simulink model "atrias_system_4khz_with_boom"  (R2016b)
settings: configuration reference "Configuration4khz" (kept outside this file)
undefined symbols (not defined in the file or in its folder): BOOM_MAX_ENCODER_TICKS, elmo_sample_time, gui_disable_cmd, gui_enable_cmd, gui_exit_cmd, gui_reset_cmd, HARD_MOTOR_POSITION_LIMITS_LOWER, HARD_MOTOR_POSITION_LIMITS_UPPER, HIP_ABS_MAX_ENCODER_TICKS, HIP_CURRENT_LIMIT, HIP_INC_MAX_ENCODER_TICKS, HIP_MOTOR_CONSTANT, HIP_MTR_GEAR_RATIO, HIP_MTR_MAX_TORQUE, LEFT_MOTOR_HIP_DIRECTION, LEG1_MOTOR_A_DIRECTION, LEG1_MOTOR_B_DIRECTION, LEG2_MOTOR_A_DIRECTION, LEG2_MOTOR_B_DIRECTION, LEG_CURRENT_LIMIT, LEG_INC_ENCODER_DIRECTION_LEFT_BACK, LEG_INC_ENCODER_DIRECTION_LEFT_FRONT, LEG_INC_ENCODER_DIRECTION_RIGHT_BACK, LEG_INC_ENCODER_DIRECTION_RIGHT_FRONT, LEG_INC_ENCODER_RAD_PER_TICK, LEG_MOTOR_CONSTANT, LEG_MTR_GEAR_RATIO, LEG_MTR_MAX_TORQUE, max_hip_velocity, max_motor_velocity, MEDULLA_ADC_MAX_VOLTS, MEDULLA_ADC_OFFSET_COUNTS, MEDULLA_STATE_ERROR, MEDULLA_STATE_HALT, MEDULLA_STATE_IDLE, MEDULLA_STATE_RESET, MEDULLA_STATE_RUN, MOTOR_POSITION_LIMITS_LOWER, MOTOR_POSITION_LIMITS_UPPER, MTR_HIP_MAX_CURRENT, MTR_MAX_CONT_CURRENT, MTR_MAX_COUNT, MTR_MAX_CURRENT, MTR_MAX_TEMP, RIGHT_MOTOR_HIP_DIRECTION
libraries: xpcethercatlib x203, simulink x38
(part 2 of 4)

== system atrias_system_4khz_with_boom/Ramp Velocity Commands ==
  note: For GUI
  is_run_cmd : Inport  OutDataTypeStr=boolean  PortDimensions=1
  system time [s] : Inport  Port=2  PortDimensions=1
  velocity_cmd [rad/s] x4 : Inport  Port=3
  Constant : Constant  Value=0.1
  Enabled time : Sum  Inputs=-+
  Hold Start Time : Subsystem  TreatAsAtomicUnit=on
  NOT : Logic  Operator=NOT  IconShape=distinctive  AllPortsSameDT=off  OutDataTypeStr=boolean
  Ramp Rate (Units/sec) : Gain  Gain=1/4
  Scaling Factor : Saturate  UpperLimit=1  LowerLimit=0
  Startup Ramp : Product
  Sum : Sum  Inputs=|-+
  Terminator : Terminator
  is_start_done_cmp : RelationalOperator  Operator=>  OutDataTypeStr=boolean  RndMeth=Nearest
  velocity_cmd_scaled [rad/s] x4 : Outport  OutDataTypeStr=double  PortDimensions=4
  wires:
  is_start_done_cmp/1 -> Terminator/1
  Sum/1 -> is_start_done_cmp/1
  velocity_cmd [rad/s] x4/1 -> Startup Ramp/2
  Startup Ramp/1 -> velocity_cmd_scaled [rad/s] x4/1
  Scaling Factor/1 -> Startup Ramp/1, is_start_done_cmp/2
  Ramp Rate (Units/sec)/1 -> Sum/2, Scaling Factor/1
  Enabled time/1 -> Ramp Rate (Units/sec)/1
  Hold Start Time/1(Time Out) -> Enabled time/1
  system time [s]/1 -> Enabled time/2, Hold Start Time/1(Time In)
  is_run_cmd/1 -> NOT/1
  NOT/1 -> Hold Start Time/Enable
  Constant/1 -> Sum/1

== system atrias_system_4khz_with_boom/Start Controller ==
  note: For GUI
  note: Input Order:
      |
      | backR
      | frontR
      | latR
      | backL
      | frontL
      | latL
  is_run_cmd : Inport  OutDataTypeStr=boolean  PortDimensions=1
  system time [s] : Inport  Port=2  PortDimensions=1
  tau_cmd_in [Nm] x6 : Inport  Port=3
  Enabled time : Sum  Inputs=-+
  Hold Start Time : Subsystem  TreatAsAtomicUnit=on
  Lateral Motor Saturation : Saturate  UpperLimit=HIP_MTR_MAX_TORQUE  LowerLimit=-HIP_MTR_MAX_TORQUE
      settings: AttributesFormatString=Top: %<UpperLimit>\nBottom: %<LowerLimit>
  NOT : Logic  Operator=NOT  IconShape=distinctive  AllPortsSameDT=off  OutDataTypeStr=boolean
  Ramp Rate (Units/sec) : Gain  Gain=.25
  Sagittal Motor Saturation : Saturate  UpperLimit=LEG_MTR_MAX_TORQUE  LowerLimit=-LEG_MTR_MAX_TORQUE
      settings: AttributesFormatString=Top: %<UpperLimit>\nBottom: %<LowerLimit>
  Scaling Factor : Saturate  UpperLimit=1  LowerLimit=0
  Selector : Selector  InputPortWidth=6  IndexOptions=Index vector (dialog)  Indices=[1 2 4 5 6 3]  OutputSizes=1
  Selector1 : Selector  InputPortWidth=6  IndexOptions=Index vector (dialog)  Indices=[1 2 3 4]  OutputSizes=1
  Selector2 : Selector  InputPortWidth=6  IndexOptions=Index vector (dialog)  Indices=[5 6]  OutputSizes=1
  Separated to Tau : Selector  InputPortWidth=6  IndexOptions=Index vector (dialog)  Indices=[1 2 6 3 4 5]  OutputSizes=1
  Startup Tau Ramp : Product
  Sum : Sum  Inputs=|-+
  Terminator : Terminator
  Vector Concatenate : Concatenate
  is_start_done_cmp : RelationalOperator  Operator=>  OutDataTypeStr=boolean  RndMeth=Nearest
  tau_cmd_out [Nm] x6 : Outport  OutDataTypeStr=double  PortDimensions=6
  wires:
  NOT/1 -> Hold Start Time/Enable
  is_run_cmd/1 -> NOT/1
  system time [s]/1 -> Enabled time/2, Hold Start Time/1(Time In)
  Hold Start Time/1(Time Out) -> Enabled time/1
  Enabled time/1 -> Ramp Rate (Units/sec)/1
  Ramp Rate (Units/sec)/1 -> Scaling Factor/1, Sum/2
  Scaling Factor/1 -> is_start_done_cmp/2, Startup Tau Ramp/1
  Startup Tau Ramp/1 -> tau_cmd_out [Nm] x6/1
  Selector2/1 -> Lateral Motor Saturation/1  "lateral"
  Selector1/1 -> Sagittal Motor Saturation/1  "sagittal"
  tau_cmd_in [Nm] x6/1 -> Selector/1
  Selector/1 -> Selector1/1, Selector2/1
  Sagittal Motor Saturation/1 -> Vector Concatenate/1
  Lateral Motor Saturation/1 -> Vector Concatenate/2
  Vector Concatenate/1 -> Separated to Tau/1
  Separated to Tau/1 -> Startup Tau Ramp/2
  Sum/1 -> is_start_done_cmp/1
  is_start_done_cmp/1 -> Terminator/1

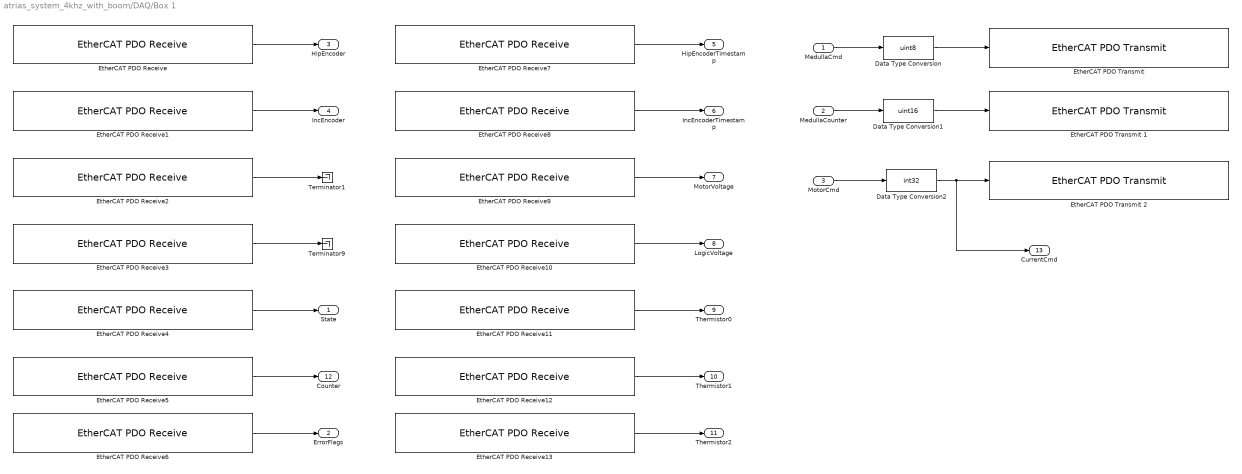
== system atrias_system_4khz_with_boom/DAQ/Box 1 ==
  MedullaCmd : Inport
  MedullaCounter : Inport  Port=2
  MotorCmd : Inport  Port=3
  Data Type Conversion : DataTypeConversion  OutDataTypeStr=uint8
  Data Type Conversion1 : DataTypeConversion  OutDataTypeStr=uint16
  Data Type Conversion2 : DataTypeConversion  OutDataTypeStr=int32
  EtherCAT PDO Receive : xpcethercatlib/EtherCAT PDO Receive  Priority=2  sig_name=Box 1 (ATRIAS 2.1 Hip (Medulla 1.5)).Hip Encoder.Encoder  sig_offset=504  sig_type=uint32  type_size=32  sig_dim=1  device_id=0  sample_time=0.001000
  EtherCAT PDO Receive1 : xpcethercatlib/EtherCAT PDO Receive  Priority=2  sig_name=Box 1 (ATRIAS 2.1 Hip (Medulla 1.5)).Incremental Encoder.Incremental Encoder  sig_offset=648  sig_type=uint16  type_size=16  sig_dim=1  device_id=0  sample_time=0.001000
  EtherCAT PDO Receive10 : xpcethercatlib/EtherCAT PDO Receive  Priority=2  sig_name=Box 1 (ATRIAS 2.1 Hip (Medulla 1.5)).Power.Logic Voltage  sig_offset=568  sig_type=uint16  type_size=16  sig_dim=1  device_id=0  sample_time=0.001000
  EtherCAT PDO Receive11 : xpcethercatlib/EtherCAT PDO Receive  Priority=2  sig_name=Box 1 (ATRIAS 2.1 Hip (Medulla 1.5)).Thermistors.Thermistor 0  sig_offset=584  sig_type=uint16  type_size=16  sig_dim=1  device_id=0  sample_time=0.001000
  EtherCAT PDO Receive12 : xpcethercatlib/EtherCAT PDO Receive  Priority=2  sig_name=Box 1 (ATRIAS 2.1 Hip (Medulla 1.5)).Thermistors.Thermistor 1  sig_offset=600  sig_type=uint16  type_size=16  sig_dim=1  device_id=0  sample_time=0.001000
  EtherCAT PDO Receive13 : xpcethercatlib/EtherCAT PDO Receive  Priority=2  sig_name=Box 1 (ATRIAS 2.1 Hip (Medulla 1.5)).Thermistors.Thermistor 2  sig_offset=616  sig_type=uint16  type_size=16  sig_dim=1  device_id=0  sample_time=0.001000
  EtherCAT PDO Receive2 : xpcethercatlib/EtherCAT PDO Receive  Priority=2  sig_name=Box 1 (ATRIAS 2.1 Hip (Medulla 1.5)).uController Status.Limit Switch  sig_offset=496  sig_type=uint8  type_size=8  sig_dim=1  device_id=0  sample_time=0.001000
  EtherCAT PDO Receive3 : xpcethercatlib/EtherCAT PDO Receive  Priority=2  sig_name=Box 1 (ATRIAS 2.1 Hip (Medulla 1.5)).uController Status.ID  sig_offset=464  sig_type=uint8  type_size=8  sig_dim=1  device_id=0  sample_time=0.001000
  EtherCAT PDO Receive4 : xpcethercatlib/EtherCAT PDO Receive  Priority=2  sig_name=Box 1 (ATRIAS 2.1 Hip (Medulla 1.5)).uController Status.State  sig_offset=472  sig_type=uint8  type_size=8  sig_dim=1  device_id=0  sample_time=0.001000
  EtherCAT PDO Receive5 : xpcethercatlib/EtherCAT PDO Receive  Priority=2  sig_name=Box 1 (ATRIAS 2.1 Hip (Medulla 1.5)).uController Status.Counter  sig_offset=480  sig_type=uint8  type_size=8  sig_dim=1  device_id=0  sample_time=0.001000
  EtherCAT PDO Receive6 : xpcethercatlib/EtherCAT PDO Receive  Priority=2  sig_name=Box 1 (ATRIAS 2.1 Hip (Medulla 1.5)).uController Status.Error Flags  sig_offset=488  sig_type=uint8  type_size=8  sig_dim=1  device_id=0  sample_time=0.001000
  EtherCAT PDO Receive7 : xpcethercatlib/EtherCAT PDO Receive  Priority=2  sig_name=Box 1 (ATRIAS 2.1 Hip (Medulla 1.5)).Hip Encoder.Timestamp  sig_offset=536  sig_type=uint16  type_size=16  sig_dim=1  device_id=0  sample_time=0.001000
  EtherCAT PDO Receive8 : xpcethercatlib/EtherCAT PDO Receive  Priority=2  sig_name=Box 1 (ATRIAS 2.1 Hip (Medulla 1.5)).Incremental Encoder.Incremental Encoder Timestamp  sig_offset=664  sig_type=uint16  type_size=16  sig_dim=1  device_id=0  sample_time=0.001000
  EtherCAT PDO Receive9 : xpcethercatlib/EtherCAT PDO Receive  Priority=2  sig_name=Box 1 (ATRIAS 2.1 Hip (Medulla 1.5)).Power.Motor Voltage  sig_offset=552  sig_type=uint16  type_size=16  sig_dim=1  device_id=0  sample_time=0.001000
  "EtherCAT PDO Transmit " : xpcethercatlib/EtherCAT PDO Transmit   Priority=3  sig_name=Box 1 (ATRIAS 2.1 Hip (Medulla 1.5)).uControllerInput.Command  sig_offset=464  sig_type=uint8  type_size=8  sig_dim=1  device_id=0  sample_time=0.001000
  EtherCAT PDO Transmit 1 : xpcethercatlib/EtherCAT PDO Transmit   Priority=3  sig_name=Box 1 (ATRIAS 2.1 Hip (Medulla 1.5)).uControllerInput.Counter  sig_offset=472  sig_type=uint16  type_size=16  sig_dim=1  device_id=0  sample_time=0.001000
  EtherCAT PDO Transmit 2 : xpcethercatlib/EtherCAT PDO Transmit   Priority=3  sig_name=Box 1 (ATRIAS 2.1 Hip (Medulla 1.5)).uControllerInput.Motor Current  sig_offset=488  sig_type=int32  type_size=32  sig_dim=1  device_id=0  sample_time=0.001000
  Terminator1 : Terminator
  Terminator9 : Terminator
  State : Outport
  ErrorFlags : Outport  Port=2
  HipEncoder : Outport  Port=3
  IncEncoder : Outport  Port=4
  HipEncoderTimestamp : Outport  Port=5
  IncEncoderTimestamp : Outport  Port=6
  MotorVoltage : Outport  Port=7
  LogicVoltage : Outport  Port=8
  Thermistor0 : Outport  Port=9
  Thermistor1 : Outport  Port=10
  Thermistor2 : Outport  Port=11
  Counter : Outport  Port=12
  CurrentCmd : Outport  Port=13
  wires:
  Data Type Conversion/1 -> "EtherCAT PDO Transmit "/1
  Data Type Conversion1/1 -> EtherCAT PDO Transmit 1/1
  Data Type Conversion2/1 -> CurrentCmd/1, EtherCAT PDO Transmit 2/1
  MedullaCmd/1 -> Data Type Conversion/1
  MedullaCounter/1 -> Data Type Conversion1/1
  MotorCmd/1 -> Data Type Conversion2/1
  EtherCAT PDO Receive8/1 -> IncEncoderTimestamp/1
  EtherCAT PDO Receive/1 -> HipEncoder/1
  EtherCAT PDO Receive7/1 -> HipEncoderTimestamp/1
  EtherCAT PDO Receive1/1 -> IncEncoder/1
  EtherCAT PDO Receive5/1 -> Counter/1
  EtherCAT PDO Receive3/1 -> Terminator9/1
  EtherCAT PDO Receive4/1 -> State/1
  EtherCAT PDO Receive6/1 -> ErrorFlags/1
  EtherCAT PDO Receive10/1 -> LogicVoltage/1
  EtherCAT PDO Receive9/1 -> MotorVoltage/1
  EtherCAT PDO Receive11/1 -> Thermistor0/1
  EtherCAT PDO Receive12/1 -> Thermistor1/1
  EtherCAT PDO Receive13/1 -> Thermistor2/1
  EtherCAT PDO Receive2/1 -> Terminator1/1

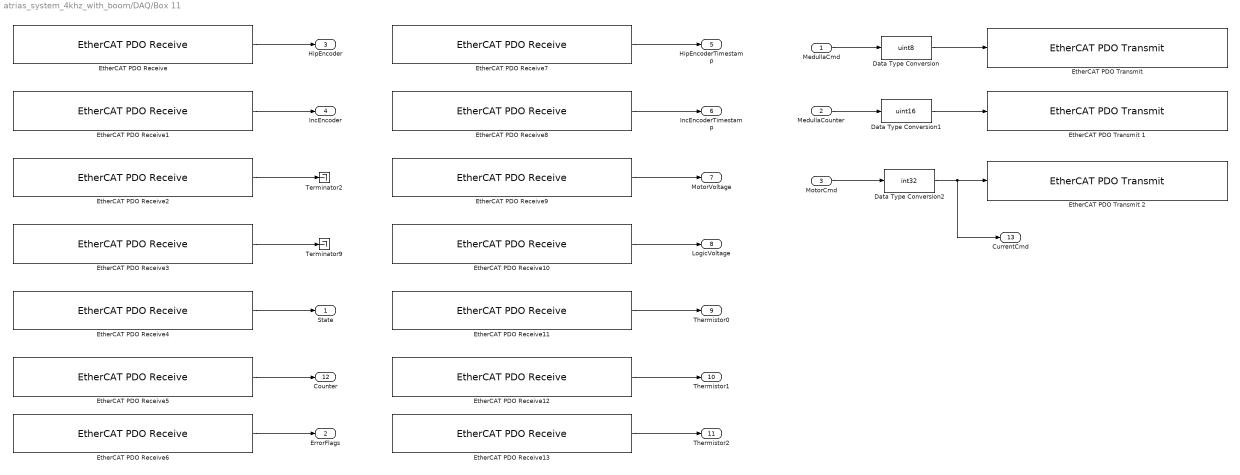
== system atrias_system_4khz_with_boom/DAQ/Box 11 ==
  MedullaCmd : Inport
  MedullaCounter : Inport  Port=2
  MotorCmd : Inport  Port=3
  Data Type Conversion : DataTypeConversion  OutDataTypeStr=uint8
  Data Type Conversion1 : DataTypeConversion  OutDataTypeStr=uint16
  Data Type Conversion2 : DataTypeConversion  OutDataTypeStr=int32
  EtherCAT PDO Receive : xpcethercatlib/EtherCAT PDO Receive  Priority=2  sig_name=Box 11 (ATRIAS 2.1 Hip (Medulla 1.5)).Hip Encoder.Encoder  sig_offset=2512  sig_type=uint32  type_size=32  sig_dim=1  device_id=0  sample_time=0.001000
  EtherCAT PDO Receive1 : xpcethercatlib/EtherCAT PDO Receive  Priority=2  sig_name=Box 11 (ATRIAS 2.1 Hip (Medulla 1.5)).Incremental Encoder.Incremental Encoder  sig_offset=2656  sig_type=uint16  type_size=16  sig_dim=1  device_id=0  sample_time=0.001000
  EtherCAT PDO Receive10 : xpcethercatlib/EtherCAT PDO Receive  Priority=2  sig_name=Box 11 (ATRIAS 2.1 Hip (Medulla 1.5)).Power.Logic Voltage  sig_offset=2576  sig_type=uint16  type_size=16  sig_dim=1  device_id=0  sample_time=0.001000
  EtherCAT PDO Receive11 : xpcethercatlib/EtherCAT PDO Receive  Priority=2  sig_name=Box 11 (ATRIAS 2.1 Hip (Medulla 1.5)).Thermistors.Thermistor 0  sig_offset=2592  sig_type=uint16  type_size=16  sig_dim=1  device_id=0  sample_time=0.001000
  EtherCAT PDO Receive12 : xpcethercatlib/EtherCAT PDO Receive  Priority=2  sig_name=Box 11 (ATRIAS 2.1 Hip (Medulla 1.5)).Thermistors.Thermistor 1  sig_offset=2608  sig_type=uint16  type_size=16  sig_dim=1  device_id=0  sample_time=0.001000
  EtherCAT PDO Receive13 : xpcethercatlib/EtherCAT PDO Receive  Priority=2  sig_name=Box 11 (ATRIAS 2.1 Hip (Medulla 1.5)).Thermistors.Thermistor 2  sig_offset=2624  sig_type=uint16  type_size=16  sig_dim=1  device_id=0  sample_time=0.001000
  EtherCAT PDO Receive2 : xpcethercatlib/EtherCAT PDO Receive  Priority=2  sig_name=Box 11 (ATRIAS 2.1 Hip (Medulla 1.5)).uController Status.Limit Switch  sig_offset=2504  sig_type=uint8  type_size=8  sig_dim=1  device_id=0  sample_time=0.001000
  EtherCAT PDO Receive3 : xpcethercatlib/EtherCAT PDO Receive  Priority=2  sig_name=Box 11 (ATRIAS 2.1 Hip (Medulla 1.5)).uController Status.ID  sig_offset=2472  sig_type=uint8  type_size=8  sig_dim=1  device_id=0  sample_time=0.001000
  EtherCAT PDO Receive4 : xpcethercatlib/EtherCAT PDO Receive  Priority=2  sig_name=Box 11 (ATRIAS 2.1 Hip (Medulla 1.5)).uController Status.State  sig_offset=2480  sig_type=uint8  type_size=8  sig_dim=1  device_id=0  sample_time=0.001000
  EtherCAT PDO Receive5 : xpcethercatlib/EtherCAT PDO Receive  Priority=2  sig_name=Box 11 (ATRIAS 2.1 Hip (Medulla 1.5)).uController Status.Counter  sig_offset=2488  sig_type=uint8  type_size=8  sig_dim=1  device_id=0  sample_time=0.001000
  EtherCAT PDO Receive6 : xpcethercatlib/EtherCAT PDO Receive  Priority=2  sig_name=Box 11 (ATRIAS 2.1 Hip (Medulla 1.5)).uController Status.Error Flags  sig_offset=2496  sig_type=uint8  type_size=8  sig_dim=1  device_id=0  sample_time=0.001000
  EtherCAT PDO Receive7 : xpcethercatlib/EtherCAT PDO Receive  Priority=2  sig_name=Box 11 (ATRIAS 2.1 Hip (Medulla 1.5)).Hip Encoder.Timestamp  sig_offset=2544  sig_type=uint16  type_size=16  sig_dim=1  device_id=0  sample_time=0.001000
  EtherCAT PDO Receive8 : xpcethercatlib/EtherCAT PDO Receive  Priority=2  sig_name=Box 11 (ATRIAS 2.1 Hip (Medulla 1.5)).Incremental Encoder.Incremental Encoder Timestamp  sig_offset=2672  sig_type=uint16  type_size=16  sig_dim=1  device_id=0  sample_time=0.001000
  EtherCAT PDO Receive9 : xpcethercatlib/EtherCAT PDO Receive  Priority=2  sig_name=Box 11 (ATRIAS 2.1 Hip (Medulla 1.5)).Power.Motor Voltage  sig_offset=2560  sig_type=uint16  type_size=16  sig_dim=1  device_id=0  sample_time=0.001000
  EtherCAT PDO Transmit : xpcethercatlib/EtherCAT PDO Transmit   Priority=3  sig_name=Box 11 (ATRIAS 2.1 Hip (Medulla 1.5)).uControllerInput.Command  sig_offset=2472  sig_type=uint8  type_size=8  sig_dim=1  device_id=0  sample_time=0.001000
  "EtherCAT PDO Transmit 1 " : xpcethercatlib/EtherCAT PDO Transmit   Priority=3  sig_name=Box 11 (ATRIAS 2.1 Hip (Medulla 1.5)).uControllerInput.Counter  sig_offset=2480  sig_type=uint16  type_size=16  sig_dim=1  device_id=0  sample_time=0.001000
  EtherCAT PDO Transmit 2 : xpcethercatlib/EtherCAT PDO Transmit   Priority=3  sig_name=Box 11 (ATRIAS 2.1 Hip (Medulla 1.5)).uControllerInput.Motor Current  sig_offset=2496  sig_type=int32  type_size=32  sig_dim=1  device_id=0  sample_time=0.001000
  Terminator2 : Terminator
  Terminator9 : Terminator
  State : Outport
  ErrorFlags : Outport  Port=2
  HipEncoder : Outport  Port=3
  IncEncoder : Outport  Port=4
  HipEncoderTimestamp : Outport  Port=5
  IncEncoderTimestamp : Outport  Port=6
  MotorVoltage : Outport  Port=7
  LogicVoltage : Outport  Port=8
  Thermistor0 : Outport  Port=9
  Thermistor1 : Outport  Port=10
  Thermistor2 : Outport  Port=11
  Counter : Outport  Port=12
  CurrentCmd : Outport  Port=13
  wires:
  Data Type Conversion/1 -> EtherCAT PDO Transmit/1
  Data Type Conversion1/1 -> "EtherCAT PDO Transmit 1 "/1
  Data Type Conversion2/1 -> CurrentCmd/1, EtherCAT PDO Transmit 2/1
  MedullaCmd/1 -> Data Type Conversion/1
  MedullaCounter/1 -> Data Type Conversion1/1
  MotorCmd/1 -> Data Type Conversion2/1
  EtherCAT PDO Receive8/1 -> IncEncoderTimestamp/1
  EtherCAT PDO Receive/1 -> HipEncoder/1
  EtherCAT PDO Receive7/1 -> HipEncoderTimestamp/1
  EtherCAT PDO Receive1/1 -> IncEncoder/1
  EtherCAT PDO Receive5/1 -> Counter/1
  EtherCAT PDO Receive3/1 -> Terminator9/1
  EtherCAT PDO Receive2/1 -> Terminator2/1
  EtherCAT PDO Receive4/1 -> State/1
  EtherCAT PDO Receive6/1 -> ErrorFlags/1
  EtherCAT PDO Receive10/1 -> LogicVoltage/1
  EtherCAT PDO Receive9/1 -> MotorVoltage/1
  EtherCAT PDO Receive11/1 -> Thermistor0/1
  EtherCAT PDO Receive12/1 -> Thermistor1/1
  EtherCAT PDO Receive13/1 -> Thermistor2/1

== system atrias_system_4khz_with_boom/DAQ/Box 2 ==
  MedullaCmd : Inport
  MedullaCounter : Inport  Port=2
  Data Type Conversion : DataTypeConversion  OutDataTypeStr=uint8
  Data Type Conversion1 : DataTypeConversion  OutDataTypeStr=uint16
  EtherCAT PDO Receive1 : xpcethercatlib/EtherCAT PDO Receive  Priority=2  sig_name=Box 12 (ATRIAS 2.1 Boom (Medulla 1.5)).X Encoder.Encoder  sig_offset=2848  sig_type=uint32  type_size=32  sig_dim=1  device_id=0  sample_time=0.001
  EtherCAT PDO Receive13 : xpcethercatlib/EtherCAT PDO Receive  Priority=2  sig_name=Box 12 (ATRIAS 2.1 Boom (Medulla 1.5)).uController Status.Counter  sig_offset=2832  sig_type=uint8  type_size=8  sig_dim=1  device_id=0  sample_time=0.001
  EtherCAT PDO Receive2 : xpcethercatlib/EtherCAT PDO Receive  Priority=2  sig_name=Box 12 (ATRIAS 2.1 Boom (Medulla 1.5)).Z Encoder.Encoder  sig_offset=2944  sig_type=uint32  type_size=32  sig_dim=1  device_id=0  sample_time=0.001
  EtherCAT PDO Receive3 : xpcethercatlib/EtherCAT PDO Receive  Priority=2  sig_name=Box 12 (ATRIAS 2.1 Boom (Medulla 1.5)).X Encoder.Timestamp  sig_offset=2880  sig_type=uint16  type_size=16  sig_dim=1  device_id=0  sample_time=0.001
  EtherCAT PDO Receive4 : xpcethercatlib/EtherCAT PDO Receive  Priority=2  sig_name=Box 12 (ATRIAS 2.1 Boom (Medulla 1.5)).Pitch Encoder.Encoder  sig_offset=2896  sig_type=uint32  type_size=32  sig_dim=1  device_id=0  sample_time=0.001
  EtherCAT PDO Receive5 : xpcethercatlib/EtherCAT PDO Receive  Priority=2  sig_name=Box 12 (ATRIAS 2.1 Boom (Medulla 1.5)).Z Encoder.Timestamp  sig_offset=2976  sig_type=uint16  type_size=16  sig_dim=1  device_id=0  sample_time=0.001
  EtherCAT PDO Receive6 : xpcethercatlib/EtherCAT PDO Receive  Priority=2  sig_name=Box 12 (ATRIAS 2.1 Boom (Medulla 1.5)).Pitch Encoder.Timestamp  sig_offset=2928  sig_type=uint16  type_size=16  sig_dim=1  device_id=0  sample_time=0.001
  EtherCAT PDO Transmit : xpcethercatlib/EtherCAT PDO Transmit   Priority=3  sig_name=Box 12 (ATRIAS 2.1 Boom (Medulla 1.5)).uControllerInput.Command  sig_offset=2816  sig_type=uint8  type_size=8  sig_dim=1  device_id=0  sample_time=0.001
  EtherCAT PDO Transmit1 : xpcethercatlib/EtherCAT PDO Transmit   Priority=3  sig_name=Box 12 (ATRIAS 2.1 Boom (Medulla 1.5)).uControllerInput.Counter  sig_offset=2824  sig_type=uint16  type_size=16  sig_dim=1  device_id=0  sample_time=0.001
  Pitch Encoder : Outport
  X Encoder : Outport  Port=2
  Z Encoder : Outport  Port=3
  Pitch Encoder Timestamp : Outport  Port=4
  X Encoder Timestamp : Outport  Port=5
  Z Encoder Timestamp : Outport  Port=6
  Counter : Outport  Port=7
  wires:
  EtherCAT PDO Receive13/1 -> Counter/1
  Data Type Conversion/1 -> EtherCAT PDO Transmit/1
  Data Type Conversion1/1 -> EtherCAT PDO Transmit1/1
  MedullaCmd/1 -> Data Type Conversion/1
  MedullaCounter/1 -> Data Type Conversion1/1
  EtherCAT PDO Receive4/1 -> Pitch Encoder/1
  EtherCAT PDO Receive1/1 -> X Encoder/1
  EtherCAT PDO Receive2/1 -> Z Encoder/1
  EtherCAT PDO Receive6/1 -> Pitch Encoder Timestamp/1
  EtherCAT PDO Receive3/1 -> X Encoder Timestamp/1
  EtherCAT PDO Receive5/1 -> Z Encoder Timestamp/1

== system atrias_system_4khz_with_boom/DAQ/Box 4 ==
  MedullaCmd : Inport
  MedullaCounter : Inport  Port=2
  Data Type Conversion : DataTypeConversion  OutDataTypeStr=uint8
  Data Type Conversion1 : DataTypeConversion  OutDataTypeStr=uint16
  EtherCAT PDO Receive1 : xpcethercatlib/EtherCAT PDO Receive  Priority=2  sig_name=Box 4 (ATRIAS 2.1 IMU (Medulla 1.5)).Rotation.Y  sig_offset=776  sig_type=single  type_size=32  sig_dim=1  device_id=0  sample_time=0.001000
  EtherCAT PDO Receive11 : xpcethercatlib/EtherCAT PDO Receive  Priority=2  sig_name=Box 4 (ATRIAS 2.1 IMU (Medulla 1.5)).uController Status.ID  sig_offset=712  sig_type=uint8  type_size=8  sig_dim=1  device_id=0  sample_time=0.001000
  EtherCAT PDO Receive12 : xpcethercatlib/EtherCAT PDO Receive  Priority=2  sig_name=Box 4 (ATRIAS 2.1 IMU (Medulla 1.5)).uController Status.State  sig_offset=720  sig_type=uint8  type_size=8  sig_dim=1  device_id=0  sample_time=0.001000
  EtherCAT PDO Receive13 : xpcethercatlib/EtherCAT PDO Receive  Priority=2  sig_name=Box 4 (ATRIAS 2.1 IMU (Medulla 1.5)).uController Status.Counter  sig_offset=728  sig_type=uint8  type_size=8  sig_dim=1  device_id=0  sample_time=0.001000
  EtherCAT PDO Receive14 : xpcethercatlib/EtherCAT PDO Receive  Priority=2  sig_name=Box 4 (ATRIAS 2.1 IMU (Medulla 1.5)).uController Status.Error Flags  sig_offset=736  sig_type=uint8  type_size=8  sig_dim=1  device_id=0  sample_time=0.001000
  EtherCAT PDO Receive2 : xpcethercatlib/EtherCAT PDO Receive  Priority=2  sig_name=Box 4 (ATRIAS 2.1 IMU (Medulla 1.5)).Rotation.Z  sig_offset=808  sig_type=single  type_size=32  sig_dim=1  device_id=0  sample_time=0.001000
  EtherCAT PDO Receive3 : xpcethercatlib/EtherCAT PDO Receive  Priority=2  sig_name=Box 4 (ATRIAS 2.1 IMU (Medulla 1.5)).Acceleration.X  sig_offset=840  sig_type=single  type_size=32  sig_dim=1  device_id=0  sample_time=0.001000
  EtherCAT PDO Receive4 : xpcethercatlib/EtherCAT PDO Receive  Priority=2  sig_name=Box 4 (ATRIAS 2.1 IMU (Medulla 1.5)).Rotation.X  sig_offset=744  sig_type=single  type_size=32  sig_dim=1  device_id=0  sample_time=0.001000
  EtherCAT PDO Receive5 : xpcethercatlib/EtherCAT PDO Receive  Priority=2  sig_name=Box 4 (ATRIAS 2.1 IMU (Medulla 1.5)).Acceleration.Y  sig_offset=872  sig_type=single  type_size=32  sig_dim=1  device_id=0  sample_time=0.001000
  EtherCAT PDO Receive6 : xpcethercatlib/EtherCAT PDO Receive  Priority=2  sig_name=Box 4 (ATRIAS 2.1 IMU (Medulla 1.5)).Acceleration.Z  sig_offset=904  sig_type=single  type_size=32  sig_dim=1  device_id=0  sample_time=0.001000
  EtherCAT PDO Receive7 : xpcethercatlib/EtherCAT PDO Receive  Priority=2  sig_name=Box 4 (ATRIAS 2.1 IMU (Medulla 1.5)).Status.Status  sig_offset=936  sig_type=uint8  type_size=8  sig_dim=1  device_id=0  sample_time=0.001000
  EtherCAT PDO Receive8 : xpcethercatlib/EtherCAT PDO Receive  Priority=2  sig_name=Box 4 (ATRIAS 2.1 IMU (Medulla 1.5)).Status.Sequence  sig_offset=944  sig_type=uint8  type_size=8  sig_dim=1  device_id=0  sample_time=0.001000
  EtherCAT PDO Receive9 : xpcethercatlib/EtherCAT PDO Receive  Priority=2  sig_name=Box 4 (ATRIAS 2.1 IMU (Medulla 1.5)).Status.Temperature  sig_offset=952  sig_type=int16  type_size=16  sig_dim=1  device_id=0  sample_time=0.001000
  EtherCAT PDO Transmit : xpcethercatlib/EtherCAT PDO Transmit   Priority=3  sig_name=Box 4 (ATRIAS 2.1 IMU (Medulla 1.5)).uControllerInput.Command  sig_offset=712  sig_type=uint8  type_size=8  sig_dim=1  device_id=0  sample_time=0.001000
  EtherCAT PDO Transmit1 : xpcethercatlib/EtherCAT PDO Transmit   Priority=3  sig_name=Box 4 (ATRIAS 2.1 IMU (Medulla 1.5)).uControllerInput.Counter  sig_offset=720  sig_type=uint16  type_size=16  sig_dim=1  device_id=0  sample_time=0.001000
  Terminator1 : Terminator
  Terminator2 : Terminator
  Terminator9 : Terminator
  ErrorFlags : Outport
  RotationX : Outport  Port=2
  RotationY : Outport  Port=3
  RotationZ : Outport  Port=4
  AccelerationX : Outport  Port=5
  AccelerationY : Outport  Port=6
  AccelerationZ : Outport  Port=7
  Sequence : Outport  Port=8
  Status : Outport  Port=9
  Counter : Outport  Port=10
  wires:
  EtherCAT PDO Receive8/1 -> Sequence/1
  EtherCAT PDO Receive7/1 -> Status/1
  EtherCAT PDO Receive6/1 -> AccelerationZ/1
  EtherCAT PDO Receive5/1 -> AccelerationY/1
  EtherCAT PDO Receive3/1 -> AccelerationX/1
  EtherCAT PDO Receive2/1 -> RotationZ/1
  EtherCAT PDO Receive1/1 -> RotationY/1
  EtherCAT PDO Receive4/1 -> RotationX/1
  MedullaCounter/1 -> Data Type Conversion1/1
  MedullaCmd/1 -> Data Type Conversion/1
  Data Type Conversion1/1 -> EtherCAT PDO Transmit1/1
  Data Type Conversion/1 -> EtherCAT PDO Transmit/1
  EtherCAT PDO Receive13/1 -> Counter/1
  EtherCAT PDO Receive14/1 -> ErrorFlags/1
  EtherCAT PDO Receive11/1 -> Terminator9/1
  EtherCAT PDO Receive12/1 -> Terminator1/1
  EtherCAT PDO Receive9/1 -> Terminator2/1

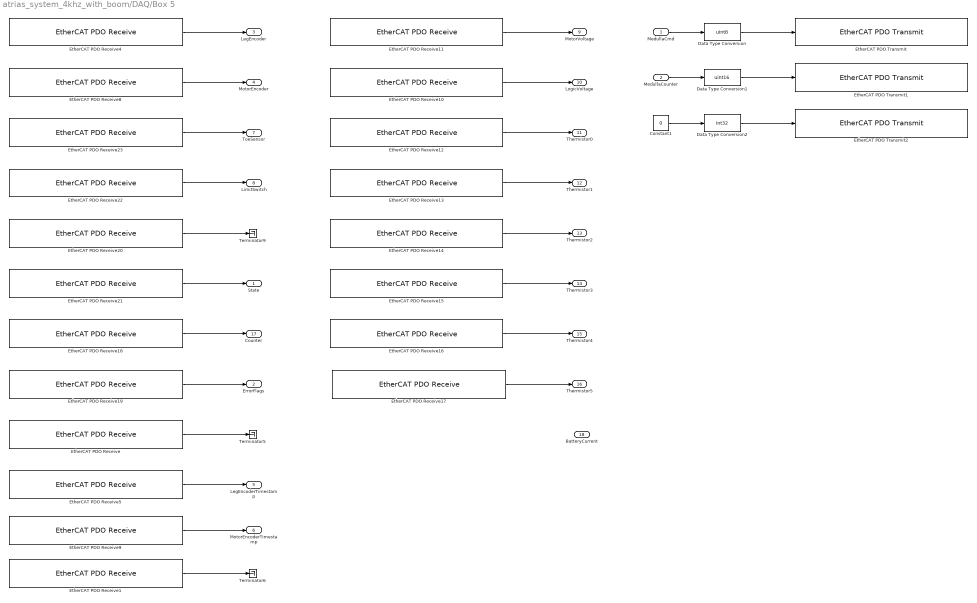
== system atrias_system_4khz_with_boom/DAQ/Box 5 ==
  MedullaCmd : Inport
  MedullaCounter : Inport  Port=2
  Constant1 : Constant  Value=0  OutDataTypeStr=Inherit: Inherit via back propagation
  Data Type Conversion : DataTypeConversion  OutDataTypeStr=uint8
  Data Type Conversion1 : DataTypeConversion  OutDataTypeStr=uint16
  Data Type Conversion2 : DataTypeConversion  OutDataTypeStr=int32
  EtherCAT PDO Receive : xpcethercatlib/EtherCAT PDO Receive  Priority=2  sig_name=Box 5 (ATRIAS 2.1 Leg (Medulla 1.5)).Incremental Encoder.Incremental Encoder  sig_offset=1120  sig_type=uint16  type_size=16  sig_dim=1  device_id=0  sample_time=0.001000
  EtherCAT PDO Receive1 : xpcethercatlib/EtherCAT PDO Receive  Priority=2  sig_name=Box 5 (ATRIAS 2.1 Leg (Medulla 1.5)).Incremental Encoder.Incremental Encoder Timestamp  sig_offset=1136  sig_type=uint16  type_size=16  sig_dim=1  device_id=0  sample_time=0.001000
  EtherCAT PDO Receive10 : xpcethercatlib/EtherCAT PDO Receive  Priority=2  sig_name=Box 5 (ATRIAS 2.1 Leg (Medulla 1.5)).Power.Logic Voltage  sig_offset=1168  sig_type=uint16  type_size=16  sig_dim=1  device_id=0  sample_time=0.001000
  EtherCAT PDO Receive11 : xpcethercatlib/EtherCAT PDO Receive  Priority=2  sig_name=Box 5 (ATRIAS 2.1 Leg (Medulla 1.5)).Power.Motor Voltage  sig_offset=1152  sig_type=uint16  type_size=16  sig_dim=1  device_id=0  sample_time=0.001000
  EtherCAT PDO Receive12 : xpcethercatlib/EtherCAT PDO Receive  Priority=2  sig_name=Box 5 (ATRIAS 2.1 Leg (Medulla 1.5)).Thermistors.Thermistor 0  sig_offset=1184  sig_type=uint16  type_size=16  sig_dim=1  device_id=0  sample_time=0.001000
  EtherCAT PDO Receive13 : xpcethercatlib/EtherCAT PDO Receive  Priority=2  sig_name=Box 5 (ATRIAS 2.1 Leg (Medulla 1.5)).Thermistors.Thermistor 1  sig_offset=1200  sig_type=uint16  type_size=16  sig_dim=1  device_id=0  sample_time=0.001000
  EtherCAT PDO Receive14 : xpcethercatlib/EtherCAT PDO Receive  Priority=2  sig_name=Box 5 (ATRIAS 2.1 Leg (Medulla 1.5)).Thermistors.Thermistor 2  sig_offset=1216  sig_type=uint16  type_size=16  sig_dim=1  device_id=0  sample_time=0.001000
  EtherCAT PDO Receive15 : xpcethercatlib/EtherCAT PDO Receive  Priority=2  sig_name=Box 5 (ATRIAS 2.1 Leg (Medulla 1.5)).Thermistors.Thermistor 3  sig_offset=1232  sig_type=uint16  type_size=16  sig_dim=1  device_id=0  sample_time=0.001000
  EtherCAT PDO Receive16 : xpcethercatlib/EtherCAT PDO Receive  Priority=2  sig_name=Box 5 (ATRIAS 2.1 Leg (Medulla 1.5)).Thermistors.Thermistor 4  sig_offset=1248  sig_type=uint16  type_size=16  sig_dim=1  device_id=0  sample_time=0.001000
  EtherCAT PDO Receive17 : xpcethercatlib/EtherCAT PDO Receive  Priority=2  sig_name=Box 5 (ATRIAS 2.1 Leg (Medulla 1.5)).Thermistors.Thermistor 5  sig_offset=1264  sig_type=uint16  type_size=16  sig_dim=1  device_id=0  sample_time=0.001000
  EtherCAT PDO Receive18 : xpcethercatlib/EtherCAT PDO Receive  Priority=2  sig_name=Box 5 (ATRIAS 2.1 Leg (Medulla 1.5)).uController Status.Counter  sig_offset=984  sig_type=uint8  type_size=8  sig_dim=1  device_id=0  sample_time=0.001000
  EtherCAT PDO Receive19 : xpcethercatlib/EtherCAT PDO Receive  Priority=2  sig_name=Box 5 (ATRIAS 2.1 Leg (Medulla 1.5)).uController Status.Error Flags  sig_offset=992  sig_type=uint8  type_size=8  sig_dim=1  device_id=0  sample_time=0.001000
  EtherCAT PDO Receive20 : xpcethercatlib/EtherCAT PDO Receive  Priority=2  sig_name=Box 5 (ATRIAS 2.1 Leg (Medulla 1.5)).uController Status.ID  sig_offset=968  sig_type=uint8  type_size=8  sig_dim=1  device_id=0  sample_time=0.001000
  EtherCAT PDO Receive21 : xpcethercatlib/EtherCAT PDO Receive  Priority=2  sig_name=Box 5 (ATRIAS 2.1 Leg (Medulla 1.5)).uController Status.State  sig_offset=976  sig_type=uint8  type_size=8  sig_dim=1  device_id=0  sample_time=0.001000
  EtherCAT PDO Receive22 : xpcethercatlib/EtherCAT PDO Receive  Priority=2  sig_name=Box 5 (ATRIAS 2.1 Leg (Medulla 1.5)).uController Status.Limit Switch  sig_offset=1000  sig_type=uint8  type_size=8  sig_dim=1  device_id=0  sample_time=0.001000
  EtherCAT PDO Receive23 : xpcethercatlib/EtherCAT PDO Receive  Priority=2  sig_name=Box 5 (ATRIAS 2.1 Leg (Medulla 1.5)).uController Status.Toe Sensor  sig_offset=1008  sig_type=uint16  type_size=16  sig_dim=1  device_id=0  sample_time=0.001000
  EtherCAT PDO Receive4 : xpcethercatlib/EtherCAT PDO Receive  Priority=2  sig_name=Box 5 (ATRIAS 2.1 Leg (Medulla 1.5)).Leg Encoder.Leg Encoder  sig_offset=1072  sig_type=uint32  type_size=32  sig_dim=1  device_id=0  sample_time=0.001000
  EtherCAT PDO Receive5 : xpcethercatlib/EtherCAT PDO Receive  Priority=2  sig_name=Box 5 (ATRIAS 2.1 Leg (Medulla 1.5)).Leg Encoder.Leg Encoder Timestamp  sig_offset=1104  sig_type=uint16  type_size=16  sig_dim=1  device_id=0  sample_time=0.001000
  EtherCAT PDO Receive8 : xpcethercatlib/EtherCAT PDO Receive  Priority=2  sig_name=Box 5 (ATRIAS 2.1 Leg (Medulla 1.5)).Motor Encoder.Motor Encoder  sig_offset=1024  sig_type=uint32  type_size=32  sig_dim=1  device_id=0  sample_time=0.001000
  EtherCAT PDO Receive9 : xpcethercatlib/EtherCAT PDO Receive  Priority=2  sig_name=Box 5 (ATRIAS 2.1 Leg (Medulla 1.5)).Motor Encoder.Motor Encoder Timestamp  sig_offset=1056  sig_type=uint16  type_size=16  sig_dim=1  device_id=0  sample_time=0.001000
  EtherCAT PDO Transmit : xpcethercatlib/EtherCAT PDO Transmit   Priority=3  sig_name=Box 5 (ATRIAS 2.1 Leg (Medulla 1.5)).uControllerInput.Command  sig_offset=968  sig_type=uint8  type_size=8  sig_dim=1  device_id=0  sample_time=0.001000
  EtherCAT PDO Transmit1 : xpcethercatlib/EtherCAT PDO Transmit   Priority=3  sig_name=Box 5 (ATRIAS 2.1 Leg (Medulla 1.5)).uControllerInput.Counter  sig_offset=976  sig_type=uint16  type_size=16  sig_dim=1  device_id=0  sample_time=0.001000
  EtherCAT PDO Transmit2 : xpcethercatlib/EtherCAT PDO Transmit   Priority=3  sig_name=Box 5 (ATRIAS 2.1 Leg (Medulla 1.5)).uControllerInput.Motor Current  sig_offset=992  sig_type=int32  type_size=32  sig_dim=1  device_id=0  sample_time=0.001000
  Terminator5 : Terminator
  Terminator6 : Terminator
  Terminator9 : Terminator
  State : Outport
  ErrorFlags : Outport  Port=2
  LegEncoder : Outport  Port=3
  MotorEncoder : Outport  Port=4
  LegEncoderTimestamp : Outport  Port=5
  MotorEncoderTimestamp : Outport  Port=6
  ToeSensor : Outport  Port=7
  LimitSwitch : Outport  Port=8
  MotorVoltage : Outport  Port=9
  LogicVoltage : Outport  Port=10
  Thermistor0 : Outport  Port=11
  Thermistor1 : Outport  Port=12
  Thermistor2 : Outport  Port=13
  Thermistor3 : Outport  Port=14
  Thermistor4 : Outport  Port=15
  Thermistor5 : Outport  Port=16
  Counter : Outport  Port=17
  BatteryCurrent : Outport  Port=18
  wires:
  Data Type Conversion1/1 -> EtherCAT PDO Transmit1/1
  EtherCAT PDO Receive/1 -> Terminator5/1
  EtherCAT PDO Receive1/1 -> Terminator6/1
  EtherCAT PDO Receive4/1 -> LegEncoder/1
  EtherCAT PDO Receive5/1 -> LegEncoderTimestamp/1
  EtherCAT PDO Receive8/1 -> MotorEncoder/1
  EtherCAT PDO Receive9/1 -> MotorEncoderTimestamp/1
  EtherCAT PDO Receive10/1 -> LogicVoltage/1
  EtherCAT PDO Receive11/1 -> MotorVoltage/1
  EtherCAT PDO Receive12/1 -> Thermistor0/1
  EtherCAT PDO Receive13/1 -> Thermistor1/1
  EtherCAT PDO Receive14/1 -> Thermistor2/1
  EtherCAT PDO Receive15/1 -> Thermistor3/1
  EtherCAT PDO Receive16/1 -> Thermistor4/1
  EtherCAT PDO Receive17/1 -> Thermistor5/1
  EtherCAT PDO Receive18/1 -> Counter/1
  EtherCAT PDO Receive19/1 -> ErrorFlags/1
  EtherCAT PDO Receive22/1 -> LimitSwitch/1
  EtherCAT PDO Receive21/1 -> State/1
  EtherCAT PDO Receive23/1 -> ToeSensor/1
  MedullaCmd/1 -> Data Type Conversion/1
  MedullaCounter/1 -> Data Type Conversion1/1
  Data Type Conversion2/1 -> EtherCAT PDO Transmit2/1
  Constant1/1 -> Data Type Conversion2/1
  EtherCAT PDO Receive20/1 -> Terminator9/1
  Data Type Conversion/1 -> EtherCAT PDO Transmit/1

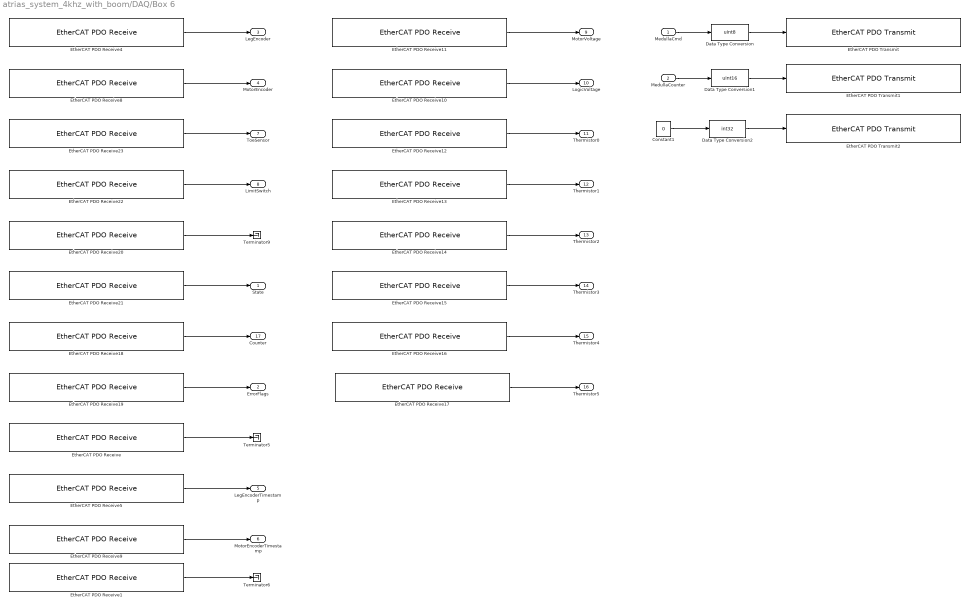
== system atrias_system_4khz_with_boom/DAQ/Box 6 ==
  MedullaCmd : Inport
  MedullaCounter : Inport  Port=2
  Constant1 : Constant  Value=0  OutDataTypeStr=Inherit: Inherit via back propagation
  Data Type Conversion : DataTypeConversion  OutDataTypeStr=uint8
  Data Type Conversion1 : DataTypeConversion  OutDataTypeStr=uint16
  Data Type Conversion2 : DataTypeConversion  OutDataTypeStr=int32
  EtherCAT PDO Receive : xpcethercatlib/EtherCAT PDO Receive  Priority=2  sig_name=Box 6 (ATRIAS 2.1 Leg (Medulla 1.5)).Incremental Encoder.Incremental Encoder  sig_offset=1496  sig_type=uint16  type_size=16  sig_dim=1  device_id=0  sample_time=0.001000
  EtherCAT PDO Receive1 : xpcethercatlib/EtherCAT PDO Receive  Priority=2  sig_name=Box 6 (ATRIAS 2.1 Leg (Medulla 1.5)).Incremental Encoder.Incremental Encoder Timestamp  sig_offset=1512  sig_type=uint16  type_size=16  sig_dim=1  device_id=0  sample_time=0.001000
  EtherCAT PDO Receive10 : xpcethercatlib/EtherCAT PDO Receive  Priority=2  sig_name=Box 6 (ATRIAS 2.1 Leg (Medulla 1.5)).Power.Logic Voltage  sig_offset=1544  sig_type=uint16  type_size=16  sig_dim=1  device_id=0  sample_time=0.001000
  EtherCAT PDO Receive11 : xpcethercatlib/EtherCAT PDO Receive  Priority=2  sig_name=Box 6 (ATRIAS 2.1 Leg (Medulla 1.5)).Power.Motor Voltage  sig_offset=1528  sig_type=uint16  type_size=16  sig_dim=1  device_id=0  sample_time=0.001000
  EtherCAT PDO Receive12 : xpcethercatlib/EtherCAT PDO Receive  Priority=2  sig_name=Box 6 (ATRIAS 2.1 Leg (Medulla 1.5)).Thermistors.Thermistor 0  sig_offset=1560  sig_type=uint16  type_size=16  sig_dim=1  device_id=0  sample_time=0.001000
  EtherCAT PDO Receive13 : xpcethercatlib/EtherCAT PDO Receive  Priority=2  sig_name=Box 6 (ATRIAS 2.1 Leg (Medulla 1.5)).Thermistors.Thermistor 1  sig_offset=1576  sig_type=uint16  type_size=16  sig_dim=1  device_id=0  sample_time=0.001000
  EtherCAT PDO Receive14 : xpcethercatlib/EtherCAT PDO Receive  Priority=2  sig_name=Box 6 (ATRIAS 2.1 Leg (Medulla 1.5)).Thermistors.Thermistor 2  sig_offset=1592  sig_type=uint16  type_size=16  sig_dim=1  device_id=0  sample_time=0.001000
  EtherCAT PDO Receive15 : xpcethercatlib/EtherCAT PDO Receive  Priority=2  sig_name=Box 6 (ATRIAS 2.1 Leg (Medulla 1.5)).Thermistors.Thermistor 3  sig_offset=1608  sig_type=uint16  type_size=16  sig_dim=1  device_id=0  sample_time=0.001000
  EtherCAT PDO Receive16 : xpcethercatlib/EtherCAT PDO Receive  Priority=2  sig_name=Box 6 (ATRIAS 2.1 Leg (Medulla 1.5)).Thermistors.Thermistor 4  sig_offset=1624  sig_type=uint16  type_size=16  sig_dim=1  device_id=0  sample_time=0.001000
  EtherCAT PDO Receive17 : xpcethercatlib/EtherCAT PDO Receive  Priority=2  sig_name=Box 6 (ATRIAS 2.1 Leg (Medulla 1.5)).Thermistors.Thermistor 5  sig_offset=1640  sig_type=uint16  type_size=16  sig_dim=1  device_id=0  sample_time=0.001000
  EtherCAT PDO Receive18 : xpcethercatlib/EtherCAT PDO Receive  Priority=2  sig_name=Box 6 (ATRIAS 2.1 Leg (Medulla 1.5)).uController Status.Counter  sig_offset=1360  sig_type=uint8  type_size=8  sig_dim=1  device_id=0  sample_time=0.001000
  EtherCAT PDO Receive19 : xpcethercatlib/EtherCAT PDO Receive  Priority=2  sig_name=Box 6 (ATRIAS 2.1 Leg (Medulla 1.5)).uController Status.Error Flags  sig_offset=1368  sig_type=uint8  type_size=8  sig_dim=1  device_id=0  sample_time=0.001000
  EtherCAT PDO Receive20 : xpcethercatlib/EtherCAT PDO Receive  Priority=2  sig_name=Box 6 (ATRIAS 2.1 Leg (Medulla 1.5)).uController Status.ID  sig_offset=1344  sig_type=uint8  type_size=8  sig_dim=1  device_id=0  sample_time=0.001000
  EtherCAT PDO Receive21 : xpcethercatlib/EtherCAT PDO Receive  Priority=2  sig_name=Box 6 (ATRIAS 2.1 Leg (Medulla 1.5)).uController Status.State  sig_offset=1352  sig_type=uint8  type_size=8  sig_dim=1  device_id=0  sample_time=0.001000
  EtherCAT PDO Receive22 : xpcethercatlib/EtherCAT PDO Receive  Priority=2  sig_name=Box 6 (ATRIAS 2.1 Leg (Medulla 1.5)).uController Status.Limit Switch  sig_offset=1376  sig_type=uint8  type_size=8  sig_dim=1  device_id=0  sample_time=0.001000
  EtherCAT PDO Receive23 : xpcethercatlib/EtherCAT PDO Receive  Priority=2  sig_name=Box 6 (ATRIAS 2.1 Leg (Medulla 1.5)).uController Status.Toe Sensor  sig_offset=1384  sig_type=uint16  type_size=16  sig_dim=1  device_id=0  sample_time=0.001000
  EtherCAT PDO Receive4 : xpcethercatlib/EtherCAT PDO Receive  Priority=2  sig_name=Box 6 (ATRIAS 2.1 Leg (Medulla 1.5)).Leg Encoder.Leg Encoder  sig_offset=1448  sig_type=uint32  type_size=32  sig_dim=1  device_id=0  sample_time=0.001000
  EtherCAT PDO Receive5 : xpcethercatlib/EtherCAT PDO Receive  Priority=2  sig_name=Box 6 (ATRIAS 2.1 Leg (Medulla 1.5)).Leg Encoder.Leg Encoder Timestamp  sig_offset=1480  sig_type=uint16  type_size=16  sig_dim=1  device_id=0  sample_time=0.001000
  EtherCAT PDO Receive8 : xpcethercatlib/EtherCAT PDO Receive  Priority=2  sig_name=Box 6 (ATRIAS 2.1 Leg (Medulla 1.5)).Motor Encoder.Motor Encoder  sig_offset=1400  sig_type=uint32  type_size=32  sig_dim=1  device_id=0  sample_time=0.001000
  EtherCAT PDO Receive9 : xpcethercatlib/EtherCAT PDO Receive  Priority=2  sig_name=Box 6 (ATRIAS 2.1 Leg (Medulla 1.5)).Motor Encoder.Motor Encoder Timestamp  sig_offset=1432  sig_type=uint16  type_size=16  sig_dim=1  device_id=0  sample_time=0.001000
  EtherCAT PDO Transmit : xpcethercatlib/EtherCAT PDO Transmit   Priority=3  sig_name=Box 6 (ATRIAS 2.1 Leg (Medulla 1.5)).uControllerInput.Command  sig_offset=1344  sig_type=uint8  type_size=8  sig_dim=1  device_id=0  sample_time=0.001000
  EtherCAT PDO Transmit1 : xpcethercatlib/EtherCAT PDO Transmit   Priority=3  sig_name=Box 6 (ATRIAS 2.1 Leg (Medulla 1.5)).uControllerInput.Counter  sig_offset=1352  sig_type=uint16  type_size=16  sig_dim=1  device_id=0  sample_time=0.001000
  EtherCAT PDO Transmit2 : xpcethercatlib/EtherCAT PDO Transmit   Priority=3  sig_name=Box 6 (ATRIAS 2.1 Leg (Medulla 1.5)).uControllerInput.Motor Current  sig_offset=1368  sig_type=int32  type_size=32  sig_dim=1  device_id=0  sample_time=0.001000
  Terminator5 : Terminator
  Terminator6 : Terminator
  Terminator9 : Terminator
  State : Outport
  ErrorFlags : Outport  Port=2
  LegEncoder : Outport  Port=3
  MotorEncoder : Outport  Port=4
  LegEncoderTimestamp : Outport  Port=5
  MotorEncoderTimestamp : Outport  Port=6
  ToeSensor : Outport  Port=7
  LimitSwitch : Outport  Port=8
  MotorVoltage : Outport  Port=9
  LogicVoltage : Outport  Port=10
  Thermistor0 : Outport  Port=11
  Thermistor1 : Outport  Port=12
  Thermistor2 : Outport  Port=13
  Thermistor3 : Outport  Port=14
  Thermistor4 : Outport  Port=15
  Thermistor5 : Outport  Port=16
  Counter : Outport  Port=17
  wires:
  Data Type Conversion/1 -> EtherCAT PDO Transmit/1
  Data Type Conversion1/1 -> EtherCAT PDO Transmit1/1
  EtherCAT PDO Receive/1 -> Terminator5/1
  EtherCAT PDO Receive1/1 -> Terminator6/1
  EtherCAT PDO Receive4/1 -> LegEncoder/1
  EtherCAT PDO Receive5/1 -> LegEncoderTimestamp/1
  EtherCAT PDO Receive8/1 -> MotorEncoder/1
  EtherCAT PDO Receive9/1 -> MotorEncoderTimestamp/1
  EtherCAT PDO Receive10/1 -> LogicVoltage/1
  EtherCAT PDO Receive11/1 -> MotorVoltage/1
  EtherCAT PDO Receive12/1 -> Thermistor0/1
  EtherCAT PDO Receive13/1 -> Thermistor1/1
  EtherCAT PDO Receive14/1 -> Thermistor2/1
  EtherCAT PDO Receive15/1 -> Thermistor3/1
  EtherCAT PDO Receive16/1 -> Thermistor4/1
  EtherCAT PDO Receive17/1 -> Thermistor5/1
  EtherCAT PDO Receive18/1 -> Counter/1
  EtherCAT PDO Receive19/1 -> ErrorFlags/1
  EtherCAT PDO Receive20/1 -> Terminator9/1
  EtherCAT PDO Receive22/1 -> LimitSwitch/1
  EtherCAT PDO Receive21/1 -> State/1
  EtherCAT PDO Receive23/1 -> ToeSensor/1
  MedullaCmd/1 -> Data Type Conversion/1
  MedullaCounter/1 -> Data Type Conversion1/1
  Data Type Conversion2/1 -> EtherCAT PDO Transmit2/1
  Constant1/1 -> Data Type Conversion2/1

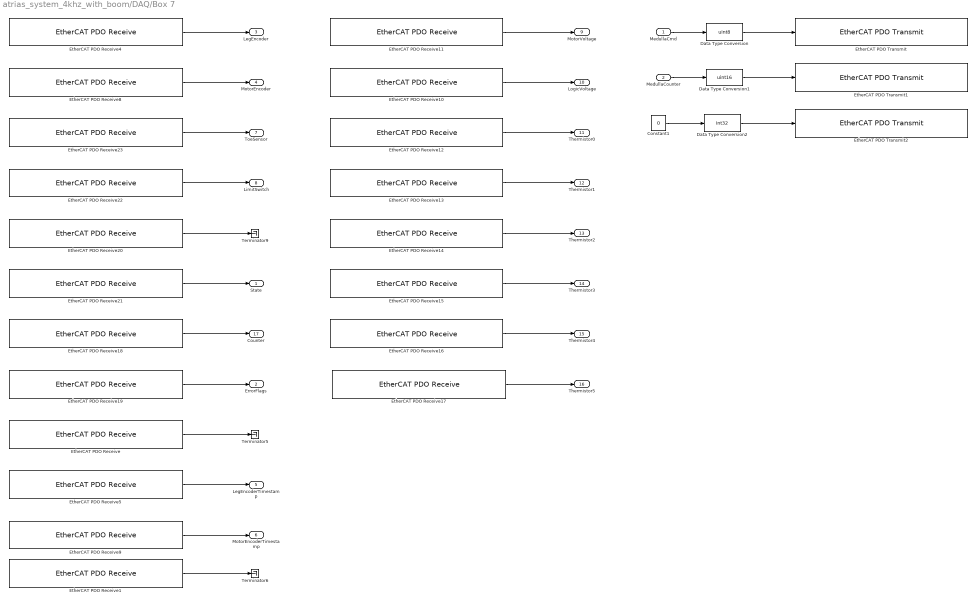
== system atrias_system_4khz_with_boom/DAQ/Box 7 ==
  MedullaCmd : Inport
  MedullaCounter : Inport  Port=2
  Constant1 : Constant  Value=0  OutDataTypeStr=Inherit: Inherit via back propagation
  Data Type Conversion : DataTypeConversion  OutDataTypeStr=uint8
  Data Type Conversion1 : DataTypeConversion  OutDataTypeStr=uint16
  Data Type Conversion2 : DataTypeConversion  OutDataTypeStr=int32
  EtherCAT PDO Receive : xpcethercatlib/EtherCAT PDO Receive  Priority=2  sig_name=Box 7 (ATRIAS 2.1 Leg (Medulla 1.5)).Incremental Encoder.Incremental Encoder  sig_offset=1872  sig_type=uint16  type_size=16  sig_dim=1  device_id=0  sample_time=0.001000
  EtherCAT PDO Receive1 : xpcethercatlib/EtherCAT PDO Receive  Priority=2  sig_name=Box 7 (ATRIAS 2.1 Leg (Medulla 1.5)).Incremental Encoder.Incremental Encoder Timestamp  sig_offset=1888  sig_type=uint16  type_size=16  sig_dim=1  device_id=0  sample_time=0.001000
  EtherCAT PDO Receive10 : xpcethercatlib/EtherCAT PDO Receive  Priority=2  sig_name=Box 7 (ATRIAS 2.1 Leg (Medulla 1.5)).Power.Logic Voltage  sig_offset=1920  sig_type=uint16  type_size=16  sig_dim=1  device_id=0  sample_time=0.001000
  EtherCAT PDO Receive11 : xpcethercatlib/EtherCAT PDO Receive  Priority=2  sig_name=Box 7 (ATRIAS 2.1 Leg (Medulla 1.5)).Power.Motor Voltage  sig_offset=1904  sig_type=uint16  type_size=16  sig_dim=1  device_id=0  sample_time=0.001000
  EtherCAT PDO Receive12 : xpcethercatlib/EtherCAT PDO Receive  Priority=2  sig_name=Box 7 (ATRIAS 2.1 Leg (Medulla 1.5)).Thermistors.Thermistor 0  sig_offset=1936  sig_type=uint16  type_size=16  sig_dim=1  device_id=0  sample_time=0.001000
  EtherCAT PDO Receive13 : xpcethercatlib/EtherCAT PDO Receive  Priority=2  sig_name=Box 7 (ATRIAS 2.1 Leg (Medulla 1.5)).Thermistors.Thermistor 1  sig_offset=1952  sig_type=uint16  type_size=16  sig_dim=1  device_id=0  sample_time=0.001000
  EtherCAT PDO Receive14 : xpcethercatlib/EtherCAT PDO Receive  Priority=2  sig_name=Box 7 (ATRIAS 2.1 Leg (Medulla 1.5)).Thermistors.Thermistor 2  sig_offset=1968  sig_type=uint16  type_size=16  sig_dim=1  device_id=0  sample_time=0.001000
  EtherCAT PDO Receive15 : xpcethercatlib/EtherCAT PDO Receive  Priority=2  sig_name=Box 7 (ATRIAS 2.1 Leg (Medulla 1.5)).Thermistors.Thermistor 3  sig_offset=1984  sig_type=uint16  type_size=16  sig_dim=1  device_id=0  sample_time=0.001000
  EtherCAT PDO Receive16 : xpcethercatlib/EtherCAT PDO Receive  Priority=2  sig_name=Box 7 (ATRIAS 2.1 Leg (Medulla 1.5)).Thermistors.Thermistor 4  sig_offset=2000  sig_type=uint16  type_size=16  sig_dim=1  device_id=0  sample_time=0.001000
  EtherCAT PDO Receive17 : xpcethercatlib/EtherCAT PDO Receive  Priority=2  sig_name=Box 7 (ATRIAS 2.1 Leg (Medulla 1.5)).Thermistors.Thermistor 5  sig_offset=2016  sig_type=uint16  type_size=16  sig_dim=1  device_id=0  sample_time=0.001000
  EtherCAT PDO Receive18 : xpcethercatlib/EtherCAT PDO Receive  Priority=2  sig_name=Box 7 (ATRIAS 2.1 Leg (Medulla 1.5)).uController Status.Counter  sig_offset=1736  sig_type=uint8  type_size=8  sig_dim=1  device_id=0  sample_time=0.001000
  EtherCAT PDO Receive19 : xpcethercatlib/EtherCAT PDO Receive  Priority=2  sig_name=Box 7 (ATRIAS 2.1 Leg (Medulla 1.5)).uController Status.Error Flags  sig_offset=1744  sig_type=uint8  type_size=8  sig_dim=1  device_id=0  sample_time=0.001000
  EtherCAT PDO Receive20 : xpcethercatlib/EtherCAT PDO Receive  Priority=2  sig_name=Box 7 (ATRIAS 2.1 Leg (Medulla 1.5)).uController Status.ID  sig_offset=1720  sig_type=uint8  type_size=8  sig_dim=1  device_id=0  sample_time=0.001000
  EtherCAT PDO Receive21 : xpcethercatlib/EtherCAT PDO Receive  Priority=2  sig_name=Box 7 (ATRIAS 2.1 Leg (Medulla 1.5)).uController Status.State  sig_offset=1728  sig_type=uint8  type_size=8  sig_dim=1  device_id=0  sample_time=0.001000
  EtherCAT PDO Receive22 : xpcethercatlib/EtherCAT PDO Receive  Priority=2  sig_name=Box 7 (ATRIAS 2.1 Leg (Medulla 1.5)).uController Status.Limit Switch  sig_offset=1752  sig_type=uint8  type_size=8  sig_dim=1  device_id=0  sample_time=0.001000
  EtherCAT PDO Receive23 : xpcethercatlib/EtherCAT PDO Receive  Priority=2  sig_name=Box 7 (ATRIAS 2.1 Leg (Medulla 1.5)).uController Status.Toe Sensor  sig_offset=1760  sig_type=uint16  type_size=16  sig_dim=1  device_id=0  sample_time=0.001000
  EtherCAT PDO Receive4 : xpcethercatlib/EtherCAT PDO Receive  Priority=2  sig_name=Box 7 (ATRIAS 2.1 Leg (Medulla 1.5)).Leg Encoder.Leg Encoder  sig_offset=1824  sig_type=uint32  type_size=32  sig_dim=1  device_id=0  sample_time=0.001000
  EtherCAT PDO Receive5 : xpcethercatlib/EtherCAT PDO Receive  Priority=2  sig_name=Box 7 (ATRIAS 2.1 Leg (Medulla 1.5)).Leg Encoder.Leg Encoder Timestamp  sig_offset=1856  sig_type=uint16  type_size=16  sig_dim=1  device_id=0  sample_time=0.001000
  EtherCAT PDO Receive8 : xpcethercatlib/EtherCAT PDO Receive  Priority=2  sig_name=Box 7 (ATRIAS 2.1 Leg (Medulla 1.5)).Motor Encoder.Motor Encoder  sig_offset=1776  sig_type=uint32  type_size=32  sig_dim=1  device_id=0  sample_time=0.001000
  EtherCAT PDO Receive9 : xpcethercatlib/EtherCAT PDO Receive  Priority=2  sig_name=Box 7 (ATRIAS 2.1 Leg (Medulla 1.5)).Motor Encoder.Motor Encoder Timestamp  sig_offset=1808  sig_type=uint16  type_size=16  sig_dim=1  device_id=0  sample_time=0.001000
  EtherCAT PDO Transmit : xpcethercatlib/EtherCAT PDO Transmit   Priority=3  sig_name=Box 7 (ATRIAS 2.1 Leg (Medulla 1.5)).uControllerInput.Command  sig_offset=1720  sig_type=uint8  type_size=8  sig_dim=1  device_id=0  sample_time=0.001000
  EtherCAT PDO Transmit1 : xpcethercatlib/EtherCAT PDO Transmit   Priority=3  sig_name=Box 7 (ATRIAS 2.1 Leg (Medulla 1.5)).uControllerInput.Counter  sig_offset=1728  sig_type=uint16  type_size=16  sig_dim=1  device_id=0  sample_time=0.001000
  EtherCAT PDO Transmit2 : xpcethercatlib/EtherCAT PDO Transmit   Priority=3  sig_name=Box 7 (ATRIAS 2.1 Leg (Medulla 1.5)).uControllerInput.Motor Current  sig_offset=1744  sig_type=int32  type_size=32  sig_dim=1  device_id=0  sample_time=0.001000
  Terminator5 : Terminator
  Terminator6 : Terminator
  Terminator9 : Terminator
  State : Outport
  ErrorFlags : Outport  Port=2
  LegEncoder : Outport  Port=3
  MotorEncoder : Outport  Port=4
  LegEncoderTimestamp : Outport  Port=5
  MotorEncoderTimestamp : Outport  Port=6
  ToeSensor : Outport  Port=7
  LimitSwitch : Outport  Port=8
  MotorVoltage : Outport  Port=9
  LogicVoltage : Outport  Port=10
  Thermistor0 : Outport  Port=11
  Thermistor1 : Outport  Port=12
  Thermistor2 : Outport  Port=13
  Thermistor3 : Outport  Port=14
  Thermistor4 : Outport  Port=15
  Thermistor5 : Outport  Port=16
  Counter : Outport  Port=17
  wires:
  Data Type Conversion1/1 -> EtherCAT PDO Transmit1/1
  EtherCAT PDO Receive/1 -> Terminator5/1
  EtherCAT PDO Receive1/1 -> Terminator6/1
  EtherCAT PDO Receive4/1 -> LegEncoder/1
  EtherCAT PDO Receive5/1 -> LegEncoderTimestamp/1
  EtherCAT PDO Receive8/1 -> MotorEncoder/1
  EtherCAT PDO Receive9/1 -> MotorEncoderTimestamp/1
  EtherCAT PDO Receive10/1 -> LogicVoltage/1
  EtherCAT PDO Receive11/1 -> MotorVoltage/1
  EtherCAT PDO Receive12/1 -> Thermistor0/1
  EtherCAT PDO Receive13/1 -> Thermistor1/1
  EtherCAT PDO Receive14/1 -> Thermistor2/1
  EtherCAT PDO Receive15/1 -> Thermistor3/1
  EtherCAT PDO Receive16/1 -> Thermistor4/1
  EtherCAT PDO Receive17/1 -> Thermistor5/1
  EtherCAT PDO Receive18/1 -> Counter/1
  EtherCAT PDO Receive19/1 -> ErrorFlags/1
  EtherCAT PDO Receive20/1 -> Terminator9/1
  EtherCAT PDO Receive22/1 -> LimitSwitch/1
  EtherCAT PDO Receive21/1 -> State/1
  EtherCAT PDO Receive23/1 -> ToeSensor/1
  MedullaCmd/1 -> Data Type Conversion/1
  MedullaCounter/1 -> Data Type Conversion1/1
  Data Type Conversion2/1 -> EtherCAT PDO Transmit2/1
  Constant1/1 -> Data Type Conversion2/1
  Data Type Conversion/1 -> EtherCAT PDO Transmit/1
